simulink model "system_model"  (Simulink 7.4)
settings: Solver=ode15s  StartTime=0.0  StopTime=20  FixedStep=.1  RelTol=1e-3
values from neighbouring files (symbols this model uses):
  da_coeff = 8.5*10^(-3)    (= 0.0085)    [a2_data_input_examsim1.m]
  dp_coeff = 6*10^(-2)    (= 0.06)    [a2_data_input_examsim1.m]
  dp_freq = 10    [a2_data_input_examsim1.m]
  dp_type = 2    [a2_data_input_examsim1.m]
  dr_coeff = 1    [a2_data_input_examsim1.m]
  dr_h = 0    [a2_data_input_examsim1.m]
  ds_coeff = 1*10^(-3)    (= 0.001)    [a2_data_input_examsim1.m]
  ds_freq = 10000    [a2_data_input_examsim1.m]
  Ga = 3    [a2_data_input_examsim1.m]
  Gd = 1    [a2_data_input_examsim1.m]
  Gf = Gr/(Kd*Gs)    [a3_process_input.m]
  Gr = 1    [a2_data_input_examsim1.m]
  Gs = 1    [a2_data_input_examsim1.m]
libraries: cstblocks x2, simulink x1
settings Model: Creator=s177063  LastModifiedBy=Vittorio
settings DataIOCC: ExternalInput=[t,u]  LimitDataPoints=off  LoadExternalInput=on  SaveOutput=off  SignalLogging=off
settings DebuggingCC: StrictBusMsg=ErrorLevel1

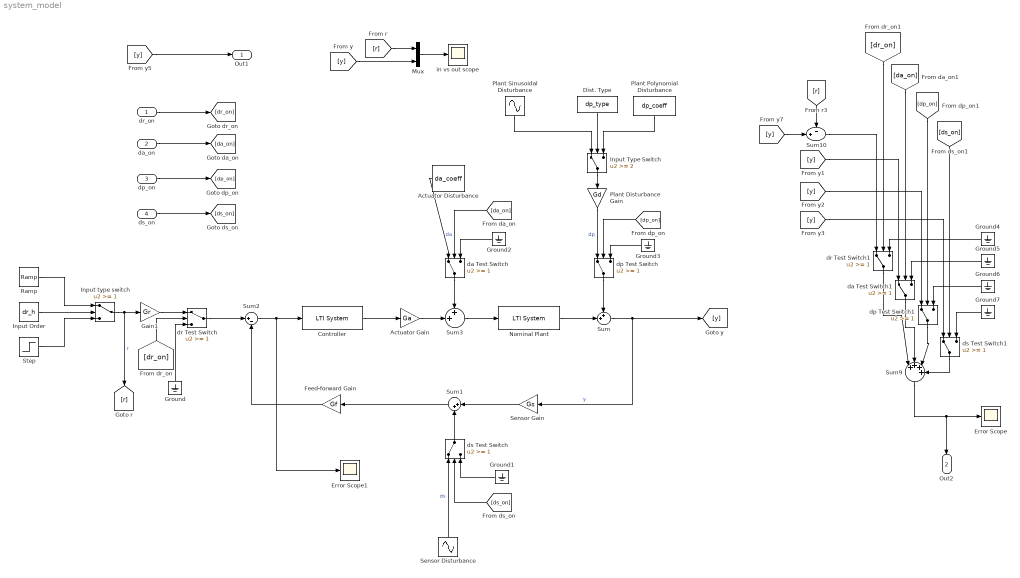
== system system_model ==
  dr_on : Inport  OutDataType=fixdt(1, 16)  OutScaling=2^0
  da_on : Inport  Port=2  OutDataType=fixdt(1, 16)  OutScaling=2^0
  dp_on : Inport  Port=3  OutDataType=fixdt(1, 16)  OutScaling=2^0
  ds_on : Inport  Port=4  OutDataType=fixdt(1, 16)  OutScaling=2^0
  Actuator Disturbance : Constant  Value=da_coeff
  Actuator Gain : Gain  Gain=Ga
  Controller : cstblocks/LTI System  SystemSampleTime=-1  sys=Gcmod  IC=[]
  Dist. Type : Constant  Value=dp_type
  Error Scope : Scope
      settings: TimeRange=0.5  YMin=0  YMax=2.5  SaveName=ScopeData3  SampleInput=on
  Error Scope1 : Scope
      settings: TimeRange=0.5  YMin=0  YMax=2.5  SampleInput=on
  Feed-forward Gain : Gain  Gain=Gf
  Gain1 : Gain  Gain=Gr
  Ground{,1..7} (8 alike) : Ground
  Input Order : Constant  Value=dr_h
  Input Type Switch : Switch  Threshold=2
  Input type switch : Switch  Threshold=1
  Mux : Mux  Inputs=2
  Nominal Plant : cstblocks/LTI System  SystemSampleTime=-1  sys=Gp_nominal  IC=[]
  Plant Disturbance Gain : Gain  Gain=Gd
  Plant Polynomial Disturbance : Constant  Value=dp_coeff
  Plant Sinusoidal Disturbance : Sin  Amplitude=dp_coeff  Bias=0  Frequency=dp_freq  Phase=0  Samples=10  SampleTime=0  Offset=0
  Ramp : simulink/Sources/Ramp  SystemSampleTime=-1  slope=dr_coeff  start=0  X0=0
  Sensor Disturbance : Sin  Amplitude=ds_coeff  Bias=0  Frequency=ds_freq  Phase=0  Samples=10  SampleTime=0  Offset=0
  Sensor Gain : Gain  Gain=Gs
  Step : Step  Time=0  After=dr_coeff  SampleTime=0
  Sum : Sum  Inputs=++|
  Sum1 : Sum  Inputs=|++
  Sum10 : Sum  Inputs=-+|
  Sum2 : Sum  Inputs=|+-
  Sum3 : Sum  Inputs=++|
  Sum9 : Sum  Inputs=|++++  OutDataType=fixdt(1, 16)  OutScaling=2^0
  da Test Switch : Switch  Threshold=1
  da Test Switch1 : Switch  Threshold=1
  dp Test Switch : Switch  Threshold=1
  dp Test Switch1 : Switch  Threshold=1
  dr Test Switch : Switch  Threshold=1
  dr Test Switch1 : Switch  Threshold=1
  ds Test Switch : Switch  Threshold=1
  ds Test Switch1 : Switch  Threshold=1
  in vs out scope : Scope
      settings: TimeRange=0.5  YMin=7.45  YMax=8.3  SampleInput=on
  Out1 : Outport  OutDataType=fixdt(1, 16)  OutScaling=2^0
  Out2 : Outport  Port=2  OutDataType=fixdt(1, 16)  OutScaling=2^0
  wires:
  Sum/1 -> Sensor Gain/1, [y]  "y"
  Controller/1 -> Actuator Gain/1
  Sum3/1 -> Nominal Plant/1
  Sum2/1 -> Controller/1, Error Scope1/1
  Sensor Gain/1 -> Sum1/1
  Sum1/1 -> Feed-forward Gain/1
  Feed-forward Gain/1 -> Sum2/2
  Actuator Gain/1 -> Sum3/2
  Nominal Plant/1 -> Sum/2
  Mux/1 -> in vs out scope/1
  Input Order/1 -> Input type switch/2
  Input type switch/1 -> Gain1/1, [r]  "r"
  Dist. Type/1 -> Input Type Switch/2
  Ramp/1 -> Input type switch/1
  Step/1 -> Input type switch/3
  Input Type Switch/1 -> Plant Disturbance Gain/1
  Plant Sinusoidal Disturbance/1 -> Input Type Switch/1
  Plant Polynomial Disturbance/1 -> Input Type Switch/3
  Plant Disturbance Gain/1 -> dp Test Switch/1  "dp"
  Sensor Disturbance/1 -> ds Test Switch/1  "ds"
  [r] -> Mux/1
  [y] -> Mux/2
  [y] -> Out1/1
  Gain1/1 -> dr Test Switch/1
  dr Test Switch/1 -> Sum2/1
  [dr_on] -> dr Test Switch/2
  da Test Switch/1 -> Sum3/1
  [da_on] -> da Test Switch/2
  ds Test Switch/1 -> Sum1/2
  dp Test Switch/1 -> Sum/1
  [dp_on] -> dp Test Switch/2
  [ds_on] -> ds Test Switch/2
  dr_on/1 -> [dr_on]
  da_on/1 -> [da_on]
  dp_on/1 -> [dp_on]
  ds_on/1 -> [ds_on]
  Sum10/1 -> dr Test Switch1/1
  [y] -> da Test Switch1/1
  [y] -> dp Test Switch1/1
  [y] -> ds Test Switch1/1
  [dr_on] -> dr Test Switch1/2
  [da_on] -> da Test Switch1/2
  [dp_on] -> dp Test Switch1/2
  [ds_on] -> ds Test Switch1/2
  dr Test Switch1/1 -> Sum9/1
  da Test Switch1/1 -> Sum9/2
  dp Test Switch1/1 -> Sum9/3
  ds Test Switch1/1 -> Sum9/4
  Ground/1 -> dr Test Switch/3
  Ground1/1 -> ds Test Switch/3
  Ground2/1 -> da Test Switch/3
  Ground3/1 -> dp Test Switch/3
  Ground4/1 -> dr Test Switch1/3
  Ground5/1 -> da Test Switch1/3
  Ground6/1 -> dp Test Switch1/3
  Ground7/1 -> ds Test Switch1/3
  [r] -> Sum10/1
  [y] -> Sum10/2
  Sum9/1 -> Error Scope/1, Out2/1
  Actuator Disturbance/1 -> da Test Switch/1  "da"
